simulink subsystem "discrete_PID_T"  (R2024b)
settings: Solver=VariableStepAuto  StartTime=0.0  StopTime=10.0  RelTol=1e-3
undefined symbols (not defined in the file or in its folder): Cd_den, Cd_num
settings Model: Creator=Riccardo Grosso  LastModifiedBy=Riccardo Grosso

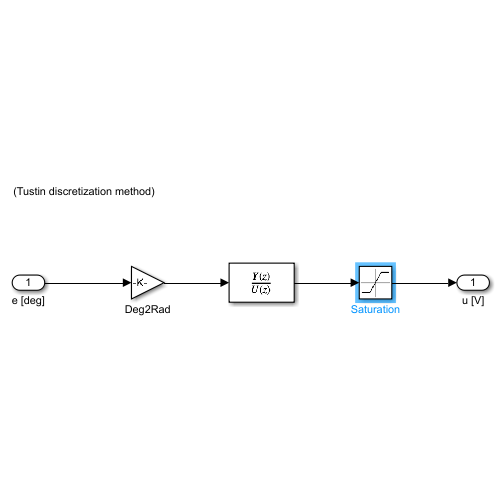
[thumbnail: Simulink's stored preview of the top-level diagram]
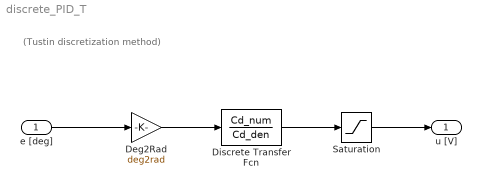
== system discrete_PID_T ==
  note: (Tustin discretization method)
  e [deg] : Inport
  Deg2Rad : Gain  Gain=deg2rad
  Discrete Transfer Fcn : DiscreteTransferFcn  Numerator=Cd_num  Denominator=Cd_den
  Saturation : Saturate  UpperLimit=12  LowerLimit=-12
  u [V] : Outport
  wires:
  e [deg]/1 -> Deg2Rad/1
  Saturation/1 -> u [V]/1
  Discrete Transfer Fcn/1 -> Saturation/1
  Deg2Rad/1 -> Discrete Transfer Fcn/1
